simulink model "a1_walking_BM"  (R2022b)
settings: Solver=VariableStepAuto  StartTime=0.0  StopTime=2  RelTol=1e-3
values from neighbouring files (symbols this model uses):
  m = 12    [MPC_Controller.m]    (also in QP_Controller.m; TASK1_rotating_mpc.m; TASK1_walking_backward_mpc.m; TASK1_walking_forward_mpc.m)
  N = 10    [MPC_Controller.m]
undefined symbols (not defined in the file or in its folder): walking_mpc, X, Y, Z
libraries: sm_lib x188, nesl_utility x108
(part 5 of 5)

== system a1_walking_BM/Rear Right Leg/Leg Logger4 ==
  PS-Simulink Converter : nesl_utility/PS-Simulink Converter  PhysicalDomain=network_engine_domain  SubClassName=ps_output  LeftPortType=input  RightPortType=output  PseudoPeriodic=off  Frequencies=[]  VectorFormat=inherit  Unit=inherit  AffineConversion=off
  PS-Simulink Converter1 : nesl_utility/PS-Simulink Converter  PhysicalDomain=network_engine_domain  SubClassName=ps_output  LeftPortType=input  RightPortType=output  PseudoPeriodic=off  Frequencies=[]  VectorFormat=inherit  Unit=inherit  AffineConversion=off
  PS-Simulink Converter2 : nesl_utility/PS-Simulink Converter  PhysicalDomain=network_engine_domain  SubClassName=ps_output  LeftPortType=input  RightPortType=output  PseudoPeriodic=off  Frequencies=[]  VectorFormat=inherit  Unit=inherit  AffineConversion=off
  Scope : Scope  NumInputPorts=3
  angle : PMIOPort  Side=Left
  velocity : PMIOPort  Port=2  Side=Left
  torque : PMIOPort  Port=3  Side=Left
  wires:
  PS-Simulink Converter/1 -> Scope/1  "RR_thigh_joint angle (rad)"
  PS-Simulink Converter2/1 -> Scope/3  "RR_thigh_joint torque (Nm)"
  PS-Simulink Converter1/1 -> Scope/2  "RR_thigh_joint velocity (rad/s)"
  connections:
  PS-Simulink Converter2/LConn1 -- torque/RConn1
  PS-Simulink Converter/LConn1 -- angle/RConn1
  PS-Simulink Converter1/LConn1 -- velocity/RConn1

== system a1_walking_BM/Rear Right Leg/RR_calf ==
  Inertia : sm_lib/Body Elements/Inertia  InertiaType=Custom  Mass=0.166  MassUnits=kg  CenterOfMass=[0, 0, 0]  CenterOfMassUnits=m  MomentsOfInertia=[0.002997972, 0.003014022, 3.2426e-05]  MomentsOfInertiaUnits=kg*m^2  ProductsOfInertia=[0, -0.000141163, 0]  ProductsOfInertiaUnits=kg*m^2  GraphicType=None  MarkerShape=Inertia  MarkerSize=20  GraphicVisPropType=SimpleVisualProperties  GraphicDiffuseColor=[0.5 0.5 0.5]  GraphicSpecularColor=[0.5 0.5 0.5 1.0]  GraphicAmbientColor=[0.15 0.15 0.15 1.0]  GraphicEmissiveColor=[0.0 0.0 0.0 1.0]  GraphicShininess=75  GraphicOpacity=1.0
  InertiaOriginTransform : sm_lib/Frames and Transforms/Rigid Transform  TranslationMethod=Cartesian  TranslationStandardOffset=0  TranslationLengthUnit=m  TranslationStandardAxis=+Z  TranslationCartesianOffset=[0.006435, 0, -0.107388]  TranslationROffset=0  TranslationROffsetUnits=m  TranslationZOffset=0  TranslationZOffsetUnits=m  TranslationThetaOffset=0  TranslationThetaOffsetUnits=deg  RotationMethod=RotationSequence  RotationAngleUnits=deg  RotationStandardAxis=+Z  RotationAngle=0.0  RotationArbitraryAxis=[0 0 1]  FollAlignAxisA=+X  BaseAlignAxisA=+Y  FollAlignAxisB=+Y  BaseAlignAxisB=+Z  RotationSequenceAxes=BaseAxes  RotationSequence=XYZ  RotationSequenceAngles=[0, 0, 0]  RotationSequenceAnglesUnits=rad  RotationMatrix=[1 0 0; 0 1 0; 0 0 1]  Quaternion=[1 0 0 0]
  RR_calf_joint_AxisInvTransform : sm_lib/Frames and Transforms/Rigid Transform  TranslationMethod=Cartesian  TranslationStandardOffset=0  TranslationLengthUnit=m  TranslationStandardAxis=+Z  TranslationCartesianOffset=[0, 0, 0]  TranslationROffset=0  TranslationROffsetUnits=m  TranslationZOffset=0  TranslationZOffsetUnits=m  TranslationThetaOffset=0  TranslationThetaOffsetUnits=deg  RotationMethod=ArbitraryAxis  RotationAngleUnits=rad  RotationStandardAxis=+Z  RotationAngle=1.570796326794897  RotationArbitraryAxis=[-1, 0, 0]  FollAlignAxisA=+X  BaseAlignAxisA=+Y  FollAlignAxisB=+Y  BaseAlignAxisB=+Z  RotationSequenceAxes=FollowerAxes  RotationSequence=XYX  RotationSequenceAngles=[0 0 0]  RotationSequenceAnglesUnits=deg  RotationMatrix=[1 0 0; 0 1 0; 0 0 1]  Quaternion=[1 0 0 0]
  RR_foot_fixed_OriginTransform : sm_lib/Frames and Transforms/Rigid Transform  TranslationMethod=Cartesian  TranslationStandardOffset=0  TranslationLengthUnit=m  TranslationStandardAxis=+Z  TranslationCartesianOffset=[0, 0, -0.2]  TranslationROffset=0  TranslationROffsetUnits=m  TranslationZOffset=0  TranslationZOffsetUnits=m  TranslationThetaOffset=0  TranslationThetaOffsetUnits=deg  RotationMethod=RotationSequence  RotationAngleUnits=deg  RotationStandardAxis=+Z  RotationAngle=0.0  RotationArbitraryAxis=[0 0 1]  FollAlignAxisA=+X  BaseAlignAxisA=+Y  FollAlignAxisB=+Y  BaseAlignAxisB=+Z  RotationSequenceAxes=BaseAxes  RotationSequence=XYZ  RotationSequenceAngles=[0, 0, 0]  RotationSequenceAnglesUnits=rad  RotationMatrix=[1 0 0; 0 1 0; 0 0 1]  Quaternion=[1 0 0 0]
  ReferenceFrame : sm_lib/Frames and Transforms/Reference Frame
  Visual : sm_lib/Body Elements/File Solid  ExtGeomFileName=AME556_project/a1_description/meshes/calf.stl  UnitType=Custom  ExtGeomFileUnits=m  StepReaderType=HEX  ExportConvexHullGeometry=off  InertiaType=Custom  Mass=0  MassUnits=kg  CenterOfMass=[0, 0, 0]  CenterOfMassUnits=m  MomentsOfInertia=[0, 0, 0]  MomentsOfInertiaUnits=kg*m^2  ProductsOfInertia=[0, 0, 0]  ProductsOfInertiaUnits=kg*m^2  BasedOnType=DensityFromFile  Density=1000  DensityUnits=kg/m^3  DoExposeReferenceFrame=on  SerializedFrames=<Frames/>  GraphicType=FromGeometry  MarkerShape=Sphere  MarkerSize=10  GraphicVisPropType=SimpleVisualProperties  GraphicDiffuseColor=[1, 0.423529411765, 0.0392156862745]  GraphicSpecularColor=[0.5 0.5 0.5 1.0]  GraphicAmbientColor=[0.15 0.15 0.15 1.0]  GraphicEmissiveColor=[0.0 0.0 0.0 1.0]  GraphicShininess=75  GraphicOpacity=1
  VisualOriginTransform : sm_lib/Frames and Transforms/Rigid Transform  TranslationMethod=Cartesian  TranslationStandardOffset=0  TranslationLengthUnit=m  TranslationStandardAxis=+Z  TranslationCartesianOffset=[0, 0, 0]  TranslationROffset=0  TranslationROffsetUnits=m  TranslationZOffset=0  TranslationZOffsetUnits=m  TranslationThetaOffset=0  TranslationThetaOffsetUnits=deg  RotationMethod=RotationSequence  RotationAngleUnits=deg  RotationStandardAxis=+Z  RotationAngle=0.0  RotationArbitraryAxis=[0 0 1]  FollAlignAxisA=+X  BaseAlignAxisA=+Y  FollAlignAxisB=+Y  BaseAlignAxisB=+Z  RotationSequenceAxes=BaseAxes  RotationSequence=XYZ  RotationSequenceAngles=[0, 0, 0]  RotationSequenceAnglesUnits=rad  RotationMatrix=[1 0 0; 0 1 0; 0 0 1]  Quaternion=[1 0 0 0]
  F : PMIOPort  Side=Left
  F1 : PMIOPort  Port=2  Side=Right
  connections:
  Inertia/RConn1 -- InertiaOriginTransform/RConn1
  RR_calf_joint_AxisInvTransform/RConn1 -- F/RConn1
  RR_foot_fixed_OriginTransform/RConn1 -- F1/RConn1
  RR_calf_joint_AxisInvTransform/LConn1 -- InertiaOriginTransform/LConn1 -- ReferenceFrame/RConn1 -- VisualOriginTransform/LConn1 -- RR_foot_fixed_OriginTransform/LConn1
  Visual/RConn1 -- VisualOriginTransform/RConn1

== system a1_walking_BM/Rear Right Leg/RR_foot ==
  Inertia : sm_lib/Body Elements/Inertia  InertiaType=Custom  Mass=0.06  MassUnits=kg  CenterOfMass=[0, 0, 0]  CenterOfMassUnits=m  MomentsOfInertia=[9.6e-06, 9.6e-06, 9.6e-06]  MomentsOfInertiaUnits=kg*m^2  ProductsOfInertia=[0, 0, 0]  ProductsOfInertiaUnits=kg*m^2  GraphicType=None  MarkerShape=Inertia  MarkerSize=20  GraphicVisPropType=SimpleVisualProperties  GraphicDiffuseColor=[0.5 0.5 0.5]  GraphicSpecularColor=[0.5 0.5 0.5 1.0]  GraphicAmbientColor=[0.15 0.15 0.15 1.0]  GraphicEmissiveColor=[0.0 0.0 0.0 1.0]  GraphicShininess=75  GraphicOpacity=1.0
  InertiaOriginTransform : sm_lib/Frames and Transforms/Rigid Transform  TranslationMethod=Cartesian  TranslationStandardOffset=0  TranslationLengthUnit=m  TranslationStandardAxis=+Z  TranslationCartesianOffset=[0, 0, 0]  TranslationROffset=0  TranslationROffsetUnits=m  TranslationZOffset=0  TranslationZOffsetUnits=m  TranslationThetaOffset=0  TranslationThetaOffsetUnits=deg  RotationMethod=RotationSequence  RotationAngleUnits=deg  RotationStandardAxis=+Z  RotationAngle=0.0  RotationArbitraryAxis=[0 0 1]  FollAlignAxisA=+X  BaseAlignAxisA=+Y  FollAlignAxisB=+Y  BaseAlignAxisB=+Z  RotationSequenceAxes=BaseAxes  RotationSequence=XYZ  RotationSequenceAngles=[0, 0, 0]  RotationSequenceAnglesUnits=rad  RotationMatrix=[1 0 0; 0 1 0; 0 0 1]  Quaternion=[1 0 0 0]
  ReferenceFrame : sm_lib/Frames and Transforms/Reference Frame
  Visual : sm_lib/Body Elements/Spherical Solid  GraphicAmbientColor=[0.15 0.15 0.15 1.0]  BasedOnType=Density  CenterOfMass=[0, 0, 0]  CenterOfMassUnits=m  GraphicDiffuseColor=[1, 0.423529411765, 0.0392156862745]  Density=1000  DensityUnits=kg/m^3  DoExposeReferenceFrame=on  GraphicEmissiveColor=[0.0 0.0 0.0 1.0]  ExportEntireGeometry=on  SerializedExposedGeometries=<ExposedGeometries><ExposedGeometry><RawGeometryId>entire</RawGeometryId><ExposedGeometryId>G</ExposedGeometryId></ExposedGeometry></ExposedGeometries>  SerializedFrames=<Frames/>  MarkerShape=Sphere  MarkerSize=10  GraphicType=FromGeometry  InertiaType=Custom  Mass=0  MassUnits=kg  MomentsOfInertia=[0, 0, 0]  MomentsOfInertiaUnits=kg*m^2  GraphicOpacity=1  ProductsOfInertia=[0, 0, 0]  ProductsOfInertiaUnits=kg*m^2  GraphicShininess=75  GraphicSpecularColor=[0.5 0.5 0.5 1.0]  SphereRadius=0.01  SphereRadiusUnits=m  GraphicVisPropType=SimpleVisualProperties
  VisualOriginTransform : sm_lib/Frames and Transforms/Rigid Transform  TranslationMethod=Cartesian  TranslationStandardOffset=0  TranslationLengthUnit=m  TranslationStandardAxis=+Z  TranslationCartesianOffset=[0, 0, 0]  TranslationROffset=0  TranslationROffsetUnits=m  TranslationZOffset=0  TranslationZOffsetUnits=m  TranslationThetaOffset=0  TranslationThetaOffsetUnits=deg  RotationMethod=RotationSequence  RotationAngleUnits=deg  RotationStandardAxis=+Z  RotationAngle=0.0  RotationArbitraryAxis=[0 0 1]  FollAlignAxisA=+X  BaseAlignAxisA=+Y  FollAlignAxisB=+Y  BaseAlignAxisB=+Z  RotationSequenceAxes=BaseAxes  RotationSequence=XYZ  RotationSequenceAngles=[0, 0, 0]  RotationSequenceAnglesUnits=rad  RotationMatrix=[1 0 0; 0 1 0; 0 0 1]  Quaternion=[1 0 0 0]
  F : PMIOPort  Side=Left
  G : PMIOPort  Port=2  Side=Left
  connections:
  Inertia/RConn1 -- InertiaOriginTransform/RConn1
  ReferenceFrame/RConn1 -- InertiaOriginTransform/LConn1 -- VisualOriginTransform/LConn1 -- F/RConn1
  Visual/RConn1 -- VisualOriginTransform/RConn1
  G/RConn1 -- Visual/LConn1

== system a1_walking_BM/Rear Right Leg/RR_hip ==
  Inertia : sm_lib/Body Elements/Inertia  InertiaType=Custom  Mass=0.696  MassUnits=kg  CenterOfMass=[0, 0, 0]  CenterOfMassUnits=m  MomentsOfInertia=[0.000469246, 0.00080749, 0.000552929]  MomentsOfInertiaUnits=kg*m^2  ProductsOfInertia=[4.66e-07, 3.42e-07, -9.408999999999999e-06]  ProductsOfInertiaUnits=kg*m^2  GraphicType=None  MarkerShape=Inertia  MarkerSize=20  GraphicVisPropType=SimpleVisualProperties  GraphicDiffuseColor=[0.5 0.5 0.5]  GraphicSpecularColor=[0.5 0.5 0.5 1.0]  GraphicAmbientColor=[0.15 0.15 0.15 1.0]  GraphicEmissiveColor=[0.0 0.0 0.0 1.0]  GraphicShininess=75  GraphicOpacity=1.0
  InertiaOriginTransform : sm_lib/Frames and Transforms/Rigid Transform  TranslationMethod=Cartesian  TranslationStandardOffset=0  TranslationLengthUnit=m  TranslationStandardAxis=+Z  TranslationCartesianOffset=[0.003311, -0.000635, 3.1e-05]  TranslationROffset=0  TranslationROffsetUnits=m  TranslationZOffset=0  TranslationZOffsetUnits=m  TranslationThetaOffset=0  TranslationThetaOffsetUnits=deg  RotationMethod=RotationSequence  RotationAngleUnits=deg  RotationStandardAxis=+Z  RotationAngle=0.0  RotationArbitraryAxis=[0 0 1]  FollAlignAxisA=+X  BaseAlignAxisA=+Y  FollAlignAxisB=+Y  BaseAlignAxisB=+Z  RotationSequenceAxes=BaseAxes  RotationSequence=XYZ  RotationSequenceAngles=[0, 0, 0]  RotationSequenceAnglesUnits=rad  RotationMatrix=[1 0 0; 0 1 0; 0 0 1]  Quaternion=[1 0 0 0]
  RR_hip_fixed_OriginTransform : sm_lib/Frames and Transforms/Rigid Transform  TranslationMethod=Cartesian  TranslationStandardOffset=0  TranslationLengthUnit=m  TranslationStandardAxis=+Z  TranslationCartesianOffset=[0, -0.081, 0]  TranslationROffset=0  TranslationROffsetUnits=m  TranslationZOffset=0  TranslationZOffsetUnits=m  TranslationThetaOffset=0  TranslationThetaOffsetUnits=deg  RotationMethod=RotationSequence  RotationAngleUnits=deg  RotationStandardAxis=+Z  RotationAngle=0.0  RotationArbitraryAxis=[0 0 1]  FollAlignAxisA=+X  BaseAlignAxisA=+Y  FollAlignAxisB=+Y  BaseAlignAxisB=+Z  RotationSequenceAxes=BaseAxes  RotationSequence=XYZ  RotationSequenceAngles=[0, 0, 0]  RotationSequenceAnglesUnits=rad  RotationMatrix=[1 0 0; 0 1 0; 0 0 1]  Quaternion=[1 0 0 0]
  RR_hip_joint_AxisInvTransform : sm_lib/Frames and Transforms/Rigid Transform  TranslationMethod=Cartesian  TranslationStandardOffset=0  TranslationLengthUnit=m  TranslationStandardAxis=+Z  TranslationCartesianOffset=[0, 0, 0]  TranslationROffset=0  TranslationROffsetUnits=m  TranslationZOffset=0  TranslationZOffsetUnits=m  TranslationThetaOffset=0  TranslationThetaOffsetUnits=deg  RotationMethod=ArbitraryAxis  RotationAngleUnits=rad  RotationStandardAxis=+Z  RotationAngle=1.570796326794897  RotationArbitraryAxis=[-0, 1, 0]  FollAlignAxisA=+X  BaseAlignAxisA=+Y  FollAlignAxisB=+Y  BaseAlignAxisB=+Z  RotationSequenceAxes=FollowerAxes  RotationSequence=XYX  RotationSequenceAngles=[0 0 0]  RotationSequenceAnglesUnits=deg  RotationMatrix=[1 0 0; 0 1 0; 0 0 1]  Quaternion=[1 0 0 0]
  RR_thigh_joint_AxisTransform : sm_lib/Frames and Transforms/Rigid Transform  TranslationMethod=Cartesian  TranslationStandardOffset=0  TranslationLengthUnit=m  TranslationStandardAxis=+Z  TranslationCartesianOffset=[0, 0, 0]  TranslationROffset=0  TranslationROffsetUnits=m  TranslationZOffset=0  TranslationZOffsetUnits=m  TranslationThetaOffset=0  TranslationThetaOffsetUnits=deg  RotationMethod=ArbitraryAxis  RotationAngleUnits=rad  RotationStandardAxis=+Z  RotationAngle=1.570796326794897  RotationArbitraryAxis=[-1, 0, 0]  FollAlignAxisA=+X  BaseAlignAxisA=+Y  FollAlignAxisB=+Y  BaseAlignAxisB=+Z  RotationSequenceAxes=FollowerAxes  RotationSequence=XYX  RotationSequenceAngles=[0 0 0]  RotationSequenceAnglesUnits=deg  RotationMatrix=[1 0 0; 0 1 0; 0 0 1]  Quaternion=[1 0 0 0]
  RR_thigh_joint_OriginTransform : sm_lib/Frames and Transforms/Rigid Transform  TranslationMethod=Cartesian  TranslationStandardOffset=0  TranslationLengthUnit=m  TranslationStandardAxis=+Z  TranslationCartesianOffset=[0, -0.0838, 0]  TranslationROffset=0  TranslationROffsetUnits=m  TranslationZOffset=0  TranslationZOffsetUnits=m  TranslationThetaOffset=0  TranslationThetaOffsetUnits=deg  RotationMethod=RotationSequence  RotationAngleUnits=deg  RotationStandardAxis=+Z  RotationAngle=0.0  RotationArbitraryAxis=[0 0 1]  FollAlignAxisA=+X  BaseAlignAxisA=+Y  FollAlignAxisB=+Y  BaseAlignAxisB=+Z  RotationSequenceAxes=BaseAxes  RotationSequence=XYZ  RotationSequenceAngles=[0, 0, 0]  RotationSequenceAnglesUnits=rad  RotationMatrix=[1 0 0; 0 1 0; 0 0 1]  Quaternion=[1 0 0 0]
  ReferenceFrame : sm_lib/Frames and Transforms/Reference Frame
  Visual : sm_lib/Body Elements/File Solid  ExtGeomFileName=AME556_project/a1_description/meshes/hip.stl  UnitType=Custom  ExtGeomFileUnits=m  StepReaderType=HEX  ExportConvexHullGeometry=off  InertiaType=Custom  Mass=0  MassUnits=kg  CenterOfMass=[0, 0, 0]  CenterOfMassUnits=m  MomentsOfInertia=[0, 0, 0]  MomentsOfInertiaUnits=kg*m^2  ProductsOfInertia=[0, 0, 0]  ProductsOfInertiaUnits=kg*m^2  BasedOnType=DensityFromFile  Density=1000  DensityUnits=kg/m^3  DoExposeReferenceFrame=on  SerializedFrames=<Frames/>  GraphicType=FromGeometry  MarkerShape=Sphere  MarkerSize=10  GraphicVisPropType=SimpleVisualProperties  GraphicDiffuseColor=[1, 0.423529411765, 0.0392156862745]  GraphicSpecularColor=[0.5 0.5 0.5 1.0]  GraphicAmbientColor=[0.15 0.15 0.15 1.0]  GraphicEmissiveColor=[0.0 0.0 0.0 1.0]  GraphicShininess=75  GraphicOpacity=1
  VisualOriginTransform : sm_lib/Frames and Transforms/Rigid Transform  TranslationMethod=Cartesian  TranslationStandardOffset=0  TranslationLengthUnit=m  TranslationStandardAxis=+Z  TranslationCartesianOffset=[0, 0, 0]  TranslationROffset=0  TranslationROffsetUnits=m  TranslationZOffset=0  TranslationZOffsetUnits=m  TranslationThetaOffset=0  TranslationThetaOffsetUnits=deg  RotationMethod=RotationSequence  RotationAngleUnits=deg  RotationStandardAxis=+Z  RotationAngle=0.0  RotationArbitraryAxis=[0 0 1]  FollAlignAxisA=+X  BaseAlignAxisA=+Y  FollAlignAxisB=+Y  BaseAlignAxisB=+Z  RotationSequenceAxes=BaseAxes  RotationSequence=XYZ  RotationSequenceAngles=[3.14159265359, 3.14159265359, 0]  RotationSequenceAnglesUnits=rad  RotationMatrix=[1 0 0; 0 1 0; 0 0 1]  Quaternion=[1 0 0 0]
  F : PMIOPort  Side=Left
  F2 : PMIOPort  Port=2  Side=Right
  F1 : PMIOPort  Port=3  Side=Right
  connections:
  Inertia/RConn1 -- InertiaOriginTransform/RConn1
  RR_hip_fixed_OriginTransform/RConn1 -- F1/RConn1
  RR_hip_joint_AxisInvTransform/RConn1 -- F/RConn1
  RR_thigh_joint_AxisTransform/RConn1 -- F2/RConn1
  RR_thigh_joint_AxisTransform/LConn1 -- RR_thigh_joint_OriginTransform/RConn1
  RR_hip_fixed_OriginTransform/LConn1 -- RR_hip_joint_AxisInvTransform/LConn1 -- RR_thigh_joint_OriginTransform/LConn1 -- InertiaOriginTransform/LConn1 -- ReferenceFrame/RConn1 -- VisualOriginTransform/LConn1
  Visual/RConn1 -- VisualOriginTransform/RConn1

== system a1_walking_BM/Rear Right Leg/RR_thigh ==
  Inertia : sm_lib/Body Elements/Inertia  InertiaType=Custom  Mass=1.013  MassUnits=kg  CenterOfMass=[0, 0, 0]  CenterOfMassUnits=m  MomentsOfInertia=[0.005529065, 0.005139339, 0.001367788]  MomentsOfInertiaUnits=kg*m^2  ProductsOfInertia=[-2.2448e-05, 0.000343869, -4.825e-06]  ProductsOfInertiaUnits=kg*m^2  GraphicType=None  MarkerShape=Inertia  MarkerSize=20  GraphicVisPropType=SimpleVisualProperties  GraphicDiffuseColor=[0.5 0.5 0.5]  GraphicSpecularColor=[0.5 0.5 0.5 1.0]  GraphicAmbientColor=[0.15 0.15 0.15 1.0]  GraphicEmissiveColor=[0.0 0.0 0.0 1.0]  GraphicShininess=75  GraphicOpacity=1.0
  InertiaOriginTransform : sm_lib/Frames and Transforms/Rigid Transform  TranslationMethod=Cartesian  TranslationStandardOffset=0  TranslationLengthUnit=m  TranslationStandardAxis=+Z  TranslationCartesianOffset=[-0.003237, 0.022327, -0.027326]  TranslationROffset=0  TranslationROffsetUnits=m  TranslationZOffset=0  TranslationZOffsetUnits=m  TranslationThetaOffset=0  TranslationThetaOffsetUnits=deg  RotationMethod=RotationSequence  RotationAngleUnits=deg  RotationStandardAxis=+Z  RotationAngle=0.0  RotationArbitraryAxis=[0 0 1]  FollAlignAxisA=+X  BaseAlignAxisA=+Y  FollAlignAxisB=+Y  BaseAlignAxisB=+Z  RotationSequenceAxes=BaseAxes  RotationSequence=XYZ  RotationSequenceAngles=[0, 0, 0]  RotationSequenceAnglesUnits=rad  RotationMatrix=[1 0 0; 0 1 0; 0 0 1]  Quaternion=[1 0 0 0]
  RR_calf_joint_AxisTransform : sm_lib/Frames and Transforms/Rigid Transform  TranslationMethod=Cartesian  TranslationStandardOffset=0  TranslationLengthUnit=m  TranslationStandardAxis=+Z  TranslationCartesianOffset=[0, 0, 0]  TranslationROffset=0  TranslationROffsetUnits=m  TranslationZOffset=0  TranslationZOffsetUnits=m  TranslationThetaOffset=0  TranslationThetaOffsetUnits=deg  RotationMethod=ArbitraryAxis  RotationAngleUnits=rad  RotationStandardAxis=+Z  RotationAngle=1.570796326794897  RotationArbitraryAxis=[-1, 0, 0]  FollAlignAxisA=+X  BaseAlignAxisA=+Y  FollAlignAxisB=+Y  BaseAlignAxisB=+Z  RotationSequenceAxes=FollowerAxes  RotationSequence=XYX  RotationSequenceAngles=[0 0 0]  RotationSequenceAnglesUnits=deg  RotationMatrix=[1 0 0; 0 1 0; 0 0 1]  Quaternion=[1 0 0 0]
  RR_calf_joint_OriginTransform : sm_lib/Frames and Transforms/Rigid Transform  TranslationMethod=Cartesian  TranslationStandardOffset=0  TranslationLengthUnit=m  TranslationStandardAxis=+Z  TranslationCartesianOffset=[0, 0, -0.2]  TranslationROffset=0  TranslationROffsetUnits=m  TranslationZOffset=0  TranslationZOffsetUnits=m  TranslationThetaOffset=0  TranslationThetaOffsetUnits=deg  RotationMethod=RotationSequence  RotationAngleUnits=deg  RotationStandardAxis=+Z  RotationAngle=0.0  RotationArbitraryAxis=[0 0 1]  FollAlignAxisA=+X  BaseAlignAxisA=+Y  FollAlignAxisB=+Y  BaseAlignAxisB=+Z  RotationSequenceAxes=BaseAxes  RotationSequence=XYZ  RotationSequenceAngles=[0, 0, 0]  RotationSequenceAnglesUnits=rad  RotationMatrix=[1 0 0; 0 1 0; 0 0 1]  Quaternion=[1 0 0 0]
  RR_thigh_joint_AxisInvTransform : sm_lib/Frames and Transforms/Rigid Transform  TranslationMethod=Cartesian  TranslationStandardOffset=0  TranslationLengthUnit=m  TranslationStandardAxis=+Z  TranslationCartesianOffset=[0, 0, 0]  TranslationROffset=0  TranslationROffsetUnits=m  TranslationZOffset=0  TranslationZOffsetUnits=m  TranslationThetaOffset=0  TranslationThetaOffsetUnits=deg  RotationMethod=ArbitraryAxis  RotationAngleUnits=rad  RotationStandardAxis=+Z  RotationAngle=1.570796326794897  RotationArbitraryAxis=[-1, 0, 0]  FollAlignAxisA=+X  BaseAlignAxisA=+Y  FollAlignAxisB=+Y  BaseAlignAxisB=+Z  RotationSequenceAxes=FollowerAxes  RotationSequence=XYX  RotationSequenceAngles=[0 0 0]  RotationSequenceAnglesUnits=deg  RotationMatrix=[1 0 0; 0 1 0; 0 0 1]  Quaternion=[1 0 0 0]
  ReferenceFrame : sm_lib/Frames and Transforms/Reference Frame
  Visual : sm_lib/Body Elements/File Solid  ExtGeomFileName=AME556_project/a1_description/meshes/thigh_mirror.stl  UnitType=Custom  ExtGeomFileUnits=m  StepReaderType=HEX  ExportConvexHullGeometry=on  InertiaType=Custom  Mass=0  MassUnits=kg  CenterOfMass=[0, 0, 0]  CenterOfMassUnits=m  MomentsOfInertia=[0, 0, 0]  MomentsOfInertiaUnits=kg*m^2  ProductsOfInertia=[0, 0, 0]  ProductsOfInertiaUnits=kg*m^2  BasedOnType=DensityFromFile  Density=1000  DensityUnits=kg/m^3  DoExposeReferenceFrame=on  SerializedFrames=<Frames/>  GraphicType=FromGeometry  MarkerShape=Sphere  MarkerSize=10  GraphicVisPropType=SimpleVisualProperties  GraphicDiffuseColor=[1, 0.423529411765, 0.0392156862745]  GraphicSpecularColor=[0.5 0.5 0.5 1.0]  GraphicAmbientColor=[0.15 0.15 0.15 1.0]  GraphicEmissiveColor=[0.0 0.0 0.0 1.0]  GraphicShininess=75  GraphicOpacity=1
  VisualOriginTransform : sm_lib/Frames and Transforms/Rigid Transform  TranslationMethod=Cartesian  TranslationStandardOffset=0  TranslationLengthUnit=m  TranslationStandardAxis=+Z  TranslationCartesianOffset=[0, 0, 0]  TranslationROffset=0  TranslationROffsetUnits=m  TranslationZOffset=0  TranslationZOffsetUnits=m  TranslationThetaOffset=0  TranslationThetaOffsetUnits=deg  RotationMethod=RotationSequence  RotationAngleUnits=deg  RotationStandardAxis=+Z  RotationAngle=0.0  RotationArbitraryAxis=[0 0 1]  FollAlignAxisA=+X  BaseAlignAxisA=+Y  FollAlignAxisB=+Y  BaseAlignAxisB=+Z  RotationSequenceAxes=BaseAxes  RotationSequence=XYZ  RotationSequenceAngles=[0, 0, 0]  RotationSequenceAnglesUnits=rad  RotationMatrix=[1 0 0; 0 1 0; 0 0 1]  Quaternion=[1 0 0 0]
  F : PMIOPort  Side=Left
  G : PMIOPort  Port=2  Side=Right
  F1 : PMIOPort  Port=3  Side=Right
  connections:
  Inertia/RConn1 -- InertiaOriginTransform/RConn1
  RR_calf_joint_AxisTransform/RConn1 -- F1/RConn1
  RR_calf_joint_AxisTransform/LConn1 -- RR_calf_joint_OriginTransform/RConn1
  RR_thigh_joint_AxisInvTransform/RConn1 -- F/RConn1
  RR_calf_joint_OriginTransform/LConn1 -- InertiaOriginTransform/LConn1 -- ReferenceFrame/RConn1 -- VisualOriginTransform/LConn1 -- RR_thigh_joint_AxisInvTransform/LConn1
  Visual/RConn1 -- VisualOriginTransform/RConn1
  G/RConn1 -- Visual/LConn1

== system a1_walking_BM/Rear Right Leg/RR_thigh_shoulder ==
  ReferenceFrame : sm_lib/Frames and Transforms/Reference Frame
  F : PMIOPort  Side=Left
  connections:
  ReferenceFrame/RConn1 -- F/RConn1

== system a1_walking_BM/Stand Controller/Subsystem1 ==
  angle : Inport
  velocity : Inport  Port=2
  Add : Sum
  Constant1 : Constant  Value=-2
  Constant2 : Constant  Value=-20
  Constant3 : Constant  Value=0.5
  Product : Product
  Product1 : Product
  Saturation : Saturate  UpperLimit=33.5  LowerLimit=-33.5
  Subtract : Sum  Inputs=+-
  Torque : Outport
  wires:
  angle/1 -> Subtract/1
  Constant2/1 -> Product/2
  Subtract/1 -> Product/1
  Constant1/1 -> Product1/2
  velocity/1 -> Product1/1
  Product1/1 -> Add/2
  Product/1 -> Add/1
  Constant3/1 -> Subtract/2
  Add/1 -> Saturation/1
  Saturation/1 -> Torque/1

== system a1_walking_BM/Stand Controller/Subsystem10 ==
  angle : Inport
  velocity : Inport  Port=2
  Add : Sum
  Constant1 : Constant  Value=-6
  Constant2 : Constant  Value=-60
  Constant3 : Constant  Value=0.8
  Product : Product
  Product1 : Product
  Saturation : Saturate  UpperLimit=33.5  LowerLimit=-33.5
  Subtract : Sum  Inputs=+-
  Torque : Outport
  wires:
  angle/1 -> Subtract/1
  Constant2/1 -> Product/2
  Subtract/1 -> Product/1
  Constant1/1 -> Product1/2
  velocity/1 -> Product1/1
  Product1/1 -> Add/2
  Product/1 -> Add/1
  Constant3/1 -> Subtract/2
  Add/1 -> Saturation/1
  Saturation/1 -> Torque/1

== system a1_walking_BM/Stand Controller/Subsystem11 ==
  angle : Inport
  velocity : Inport  Port=2
  Add : Sum
  Constant1 : Constant  Value=-4
  Constant2 : Constant  Value=-40
  Constant3 : Constant  Value=-1
  Product : Product
  Product1 : Product
  Saturation : Saturate  UpperLimit=33.5  LowerLimit=-33.5
  Subtract : Sum  Inputs=+-
  Torque : Outport
  wires:
  angle/1 -> Subtract/1
  Constant2/1 -> Product/2
  Subtract/1 -> Product/1
  Constant1/1 -> Product1/2
  velocity/1 -> Product1/1
  Product1/1 -> Add/2
  Product/1 -> Add/1
  Constant3/1 -> Subtract/2
  Add/1 -> Saturation/1
  Saturation/1 -> Torque/1

== system a1_walking_BM/Stand Controller/Subsystem12 ==
  angle : Inport
  velocity : Inport  Port=2
  Add : Sum
  Constant1 : Constant  Value=-2
  Constant2 : Constant  Value=-20
  Constant3 : Constant  Value=0
  Product : Product
  Product1 : Product
  Saturation : Saturate  UpperLimit=33.5  LowerLimit=-33.5
  Subtract : Sum  Inputs=+-
  Torque : Outport
  wires:
  angle/1 -> Subtract/1
  Constant2/1 -> Product/2
  Subtract/1 -> Product/1
  Constant1/1 -> Product1/2
  velocity/1 -> Product1/1
  Product1/1 -> Add/2
  Product/1 -> Add/1
  Constant3/1 -> Subtract/2
  Add/1 -> Saturation/1
  Saturation/1 -> Torque/1

== system a1_walking_BM/Stand Controller/Subsystem2 ==
  angle : Inport
  velocity : Inport  Port=2
  Add : Sum
  Constant1 : Constant  Value=-6
  Constant2 : Constant  Value=-60
  Constant3 : Constant  Value=0.8
  Product : Product
  Product1 : Product
  Saturation : Saturate  UpperLimit=33.5  LowerLimit=-33.5
  Subtract : Sum  Inputs=+-
  Torque : Outport
  wires:
  angle/1 -> Subtract/1
  Constant2/1 -> Product/2
  Subtract/1 -> Product/1
  Constant1/1 -> Product1/2
  velocity/1 -> Product1/1
  Product1/1 -> Add/2
  Product/1 -> Add/1
  Constant3/1 -> Subtract/2
  Add/1 -> Saturation/1
  Saturation/1 -> Torque/1

== system a1_walking_BM/Stand Controller/Subsystem3 ==
  angle : Inport
  velocity : Inport  Port=2
  Add : Sum
  Constant1 : Constant  Value=-2
  Constant2 : Constant  Value=-20
  Constant3 : Constant  Value=-1
  Product : Product
  Product1 : Product
  Saturation : Saturate  UpperLimit=33.5  LowerLimit=-33.5
  Subtract : Sum  Inputs=+-
  Torque : Outport
  wires:
  angle/1 -> Subtract/1
  Constant2/1 -> Product/2
  Subtract/1 -> Product/1
  Constant1/1 -> Product1/2
  velocity/1 -> Product1/1
  Product1/1 -> Add/2
  Product/1 -> Add/1
  Constant3/1 -> Subtract/2
  Add/1 -> Saturation/1
  Saturation/1 -> Torque/1

== system a1_walking_BM/Stand Controller/Subsystem4 ==
  angle : Inport
  velocity : Inport  Port=2
  Add : Sum
  Constant1 : Constant  Value=-4
  Constant2 : Constant  Value=-40
  Constant3 : Constant  Value=-1
  Product : Product
  Product1 : Product
  Saturation : Saturate  UpperLimit=33.5  LowerLimit=-33.5
  Subtract : Sum  Inputs=+-
  Torque : Outport
  wires:
  angle/1 -> Subtract/1
  Constant2/1 -> Product/2
  Subtract/1 -> Product/1
  Constant1/1 -> Product1/2
  velocity/1 -> Product1/1
  Product1/1 -> Add/2
  Product/1 -> Add/1
  Constant3/1 -> Subtract/2
  Add/1 -> Saturation/1
  Saturation/1 -> Torque/1

== system a1_walking_BM/Stand Controller/Subsystem5 ==
  angle : Inport
  velocity : Inport  Port=2
  Add : Sum
  Constant1 : Constant  Value=-0.5
  Constant2 : Constant  Value=-5
  Constant3 : Constant  Value=0
  Product : Product
  Product1 : Product
  Saturation : Saturate  UpperLimit=33.5  LowerLimit=-33.5
  Subtract : Sum  Inputs=+-
  Torque : Outport
  wires:
  angle/1 -> Subtract/1
  Constant2/1 -> Product/2
  Subtract/1 -> Product/1
  Constant1/1 -> Product1/2
  velocity/1 -> Product1/1
  Product1/1 -> Add/2
  Product/1 -> Add/1
  Constant3/1 -> Subtract/2
  Add/1 -> Saturation/1
  Saturation/1 -> Torque/1

== system a1_walking_BM/Stand Controller/Subsystem6 ==
  angle : Inport
  velocity : Inport  Port=2
  Add : Sum
  Constant1 : Constant  Value=-2
  Constant2 : Constant  Value=-20
  Constant3 : Constant  Value=0
  Product : Product
  Product1 : Product
  Saturation : Saturate  UpperLimit=33.5  LowerLimit=-33.5
  Subtract : Sum  Inputs=+-
  Torque : Outport
  wires:
  angle/1 -> Subtract/1
  Constant2/1 -> Product/2
  Subtract/1 -> Product/1
  Constant1/1 -> Product1/2
  velocity/1 -> Product1/1
  Product1/1 -> Add/2
  Product/1 -> Add/1
  Constant3/1 -> Subtract/2
  Add/1 -> Saturation/1
  Saturation/1 -> Torque/1

== system a1_walking_BM/Stand Controller/Subsystem7 ==
  angle : Inport
  velocity : Inport  Port=2
  Add : Sum
  Constant1 : Constant  Value=-2
  Constant2 : Constant  Value=-20
  Constant3 : Constant  Value=0.5
  Product : Product
  Product1 : Product
  Saturation : Saturate  UpperLimit=33.5  LowerLimit=-33.5
  Subtract : Sum  Inputs=+-
  Torque : Outport
  wires:
  angle/1 -> Subtract/1
  Constant2/1 -> Product/2
  Subtract/1 -> Product/1
  Constant1/1 -> Product1/2
  velocity/1 -> Product1/1
  Product1/1 -> Add/2
  Product/1 -> Add/1
  Constant3/1 -> Subtract/2
  Add/1 -> Saturation/1
  Saturation/1 -> Torque/1

== system a1_walking_BM/Stand Controller/Subsystem8 ==
  angle : Inport
  velocity : Inport  Port=2
  Add : Sum
  Constant1 : Constant  Value=-2
  Constant2 : Constant  Value=-20
  Constant3 : Constant  Value=-1
  Product : Product
  Product1 : Product
  Saturation : Saturate  UpperLimit=33.5  LowerLimit=-33.5
  Subtract : Sum  Inputs=+-
  Torque : Outport
  wires:
  angle/1 -> Subtract/1
  Constant2/1 -> Product/2
  Subtract/1 -> Product/1
  Constant1/1 -> Product1/2
  velocity/1 -> Product1/1
  Product1/1 -> Add/2
  Product/1 -> Add/1
  Constant3/1 -> Subtract/2
  Add/1 -> Saturation/1
  Saturation/1 -> Torque/1

== system a1_walking_BM/Stand Controller/Subsystem9 ==
  angle : Inport
  velocity : Inport  Port=2
  Add : Sum
  Constant1 : Constant  Value=-0.5
  Constant2 : Constant  Value=-5
  Constant3 : Constant  Value=0
  Product : Product
  Product1 : Product
  Saturation : Saturate  UpperLimit=33.5  LowerLimit=-33.5
  Subtract : Sum  Inputs=+-
  Torque : Outport
  wires:
  angle/1 -> Subtract/1
  Constant2/1 -> Product/2
  Subtract/1 -> Product/1
  Constant1/1 -> Product1/2
  velocity/1 -> Product1/1
  Product1/1 -> Add/2
  Product/1 -> Add/1
  Constant3/1 -> Subtract/2
  Add/1 -> Saturation/1
  Saturation/1 -> Torque/1

== matlab function a1_walking_BM/Stand Controller/MATLAB Function4 ==
  data: angle_vector input; hip_angle output; thigh_angle output; calf_angle output
function [hip_angle, thigh_angle, calf_angle] = fcn(angle_vector)

hip_angle = angle_vector(1);
thigh_angle = angle_vector(2);
calf_angle = angle_vector(3);

== matlab function a1_walking_BM/Stand Controller/MATLAB Function5 ==
  data: velocity_vector input; hip_velocity output; thigh_velocity output; calf_velocity output
function [hip_velocity, thigh_velocity, calf_velocity] = fcn(velocity_vector)

hip_velocity = velocity_vector(1);
thigh_velocity = velocity_vector(2);
calf_velocity = velocity_vector(3);

== matlab function a1_walking_BM/Stand Controller/MATLAB Function6 ==
  data: angle_vector input; hip_angle output; thigh_angle output; calf_angle output
function [hip_angle, thigh_angle, calf_angle] = fcn(angle_vector)

hip_angle = angle_vector(1);
thigh_angle = angle_vector(2);
calf_angle = angle_vector(3);

== matlab function a1_walking_BM/Stand Controller/MATLAB Function7 ==
  data: velocity_vector input; hip_velocity output; thigh_velocity output; calf_velocity output
function [hip_velocity, thigh_velocity, calf_velocity] = fcn(velocity_vector)

hip_velocity = velocity_vector(1);
thigh_velocity = velocity_vector(2);
calf_velocity = velocity_vector(3);

== matlab function a1_walking_BM/Swing Controller/MATLAB Function ==
  data: v_com_vec input; F output; t input; T_stance input; v_desired input; p_hip input
function F = fcn(v_com_vec,t,T_stance,v_desired,p_hip)


%% NOTE - THIS CODE IS NOT COMPLETE YET
% Find K_step - this value can be tuned with z_com_desired
z_com_desired = 0.1;
g = 9.81;
K_step = sqrt(z_com_desired/g);

% Find P_foot_desired
p_foot_desired = p_hip+(T_stance/2)*v_com_vec+K_step*(v_com_vec-v_desired);

% Find F_swing
Kp = 1; 
Kd = 1; 
F_swing = Kp*(p_foot_desired-p_foot)+Kd*(foot_vel_desired-foot_vel)

F = v_com_vec;

== matlab function a1_walking_BM/Convert Forces to Torque/Force to Torque ==
  data: F input; Tau_RR output; RR_ang_vec input; RL_ang_vec input; FL_ang_vec input; FR_ang_vec input; Tau_FR output; Tau_FL output; Tau_RL output
function [Tau_RR,Tau_FR,Tau_FL,Tau_RL]= fcn(F,RR_ang_vec,RL_ang_vec,FL_ang_vec,FR_ang_vec)
    % TODO - Convert forces to torques using the inverse jacobian

    %% NOTE - The inverse jacobians were calculated by finding the end
    % effector position and taking the partial with respect to each joint
    % Theta 2 is the hip angle 
    % Theta 4 is the thigh angle
    % Theta 5 is the calf angle 
    a2 = 0.0838; %This is the hip length (m)
    a4 = 0.2; %This is the thigh length (m)
    a5 = 0.2; %This is the calf length (m)

    % Get forces from the force vector 
    % NOTE - VERIFY THAT THESE ARE THE CORRECT VECTORS (I am unsure)
    F_FL = F(1:3);
    F_FR = F(4:6);
    F_RL = F(7:9);
    F_RR = F(10:12);

    %% Calculate the force for the RR leg - NOTE: The right legs have the
    % same jacobians
    theta2 = RR_ang_vec(1); % RE-Define theta 2 
    theta4 = RR_ang_vec(2); % RE-Define theta 4
    theta5 = RR_ang_vec(3); % RE-Define theta 5
    inJ_R_RR = [                                                                       0, a2*sin(theta2) + a4*cos(theta2)*cos(theta4) + a5*cos(theta2)*cos(theta4)*cos(theta5) - a5*cos(theta2)*sin(theta4)*sin(theta5), a4*cos(theta4)*sin(theta2) - a2*cos(theta2) + a5*cos(theta4)*cos(theta5)*sin(theta2) - a5*sin(theta2)*sin(theta4)*sin(theta5);
    a5*sin(theta4)*sin(theta5) - a5*cos(theta4)*cos(theta5) - a4*cos(theta4),                - a4*sin(theta2)*sin(theta4) - a5*cos(theta4)*sin(theta2)*sin(theta5) - a5*cos(theta5)*sin(theta2)*sin(theta4),                  a4*cos(theta2)*sin(theta4) + a5*cos(theta2)*cos(theta4)*sin(theta5) + a5*cos(theta2)*cos(theta5)*sin(theta4);
                     a5*sin(theta4)*sin(theta5) - a5*cos(theta4)*cos(theta5),                                             - a5*cos(theta4)*sin(theta2)*sin(theta5) - a5*cos(theta5)*sin(theta2)*sin(theta4),                                               a5*cos(theta2)*cos(theta4)*sin(theta5) + a5*cos(theta2)*cos(theta5)*sin(theta4)];
     
    Tau_RR = -inJ_R_RR*F_RR;

    %% Calculate the force for the FR leg - NOTE: The right legs have the
    % same jacobians
    theta2 = FR_ang_vec(1); % RE-Define theta 2 
    theta4 = FR_ang_vec(2); % RE-Define theta 4
    theta5 = FR_ang_vec(3); % RE-Define theta 5
    inJ_R_FR = [                                                                       0, a2*sin(theta2) + a4*cos(theta2)*cos(theta4) + a5*cos(theta2)*cos(theta4)*cos(theta5) - a5*cos(theta2)*sin(theta4)*sin(theta5), a4*cos(theta4)*sin(theta2) - a2*cos(theta2) + a5*cos(theta4)*cos(theta5)*sin(theta2) - a5*sin(theta2)*sin(theta4)*sin(theta5);
    a5*sin(theta4)*sin(theta5) - a5*cos(theta4)*cos(theta5) - a4*cos(theta4),                - a4*sin(theta2)*sin(theta4) - a5*cos(theta4)*sin(theta2)*sin(theta5) - a5*cos(theta5)*sin(theta2)*sin(theta4),                  a4*cos(theta2)*sin(theta4) + a5*cos(theta2)*cos(theta4)*sin(theta5) + a5*cos(theta2)*cos(theta5)*sin(theta4);
                     a5*sin(theta4)*sin(theta5) - a5*cos(theta4)*cos(theta5),                                             - a5*cos(theta4)*sin(theta2)*sin(theta5) - a5*cos(theta5)*sin(theta2)*sin(theta4),                                               a5*cos(theta2)*cos(theta4)*sin(theta5) + a5*cos(theta2)*cos(theta5)*sin(theta4)];
     
    Tau_FR = -inJ_R_FR*F_FR;

    %% Calculate the force for the FL leg - NOTE: The right legs have the
    % same jacobians
    theta2 = FL_ang_vec(1); % RE-Define theta 2 
    theta4 = FL_ang_vec(2); % RE-Define theta 4
    theta5 = FL_ang_vec(3); % RE-Define theta 5
    inJ_L_FL = [                                                                       0, a4*cos(theta2)*cos(theta4) - a2*sin(theta2) + a5*cos(theta2)*cos(theta4)*cos(theta5) - a5*cos(theta2)*sin(theta4)*sin(theta5), a2*cos(theta2) + a4*cos(theta4)*sin(theta2) + a5*cos(theta4)*cos(theta5)*sin(theta2) - a5*sin(theta2)*sin(theta4)*sin(theta5);
    a5*sin(theta4)*sin(theta5) - a5*cos(theta4)*cos(theta5) - a4*cos(theta4),                - a4*sin(theta2)*sin(theta4) - a5*cos(theta4)*sin(theta2)*sin(theta5) - a5*cos(theta5)*sin(theta2)*sin(theta4),                  a4*cos(theta2)*sin(theta4) + a5*cos(theta2)*cos(theta4)*sin(theta5) + a5*cos(theta2)*cos(theta5)*sin(theta4);
                     a5*sin(theta4)*sin(theta5) - a5*cos(theta4)*cos(theta5),                                             - a5*cos(theta4)*sin(theta2)*sin(theta5) - a5*cos(theta5)*sin(theta2)*sin(theta4),                                               a5*cos(theta2)*cos(theta4)*sin(theta5) + a5*cos(theta2)*cos(theta5)*sin(theta4)];
     
    Tau_FL = -inJ_L_FL*F_FL;


    %% Calculate the force for the RL leg - NOTE: The right legs have the
    % same jacobians
    theta2 = RL_ang_vec(1); % RE-Define theta 2 
    theta4 = RL_ang_vec(2); % RE-Define theta 4
    theta5 = RL_ang_vec(3); % RE-Define theta 5
    inJ_L_RL = [                                                                       0, a4*cos(theta2)*cos(theta4) - a2*sin(theta2) + a5*cos(theta2)*cos(theta4)*cos(theta5) - a5*cos(theta2)*sin(theta4)*sin(theta5), a2*cos(theta2) + a4*cos(theta4)*sin(theta2) + a5*cos(theta4)*cos(theta5)*sin(theta2) - a5*sin(theta2)*sin(theta4)*sin(theta5);
    a5*sin(theta4)*sin(theta5) - a5*cos(theta4)*cos(theta5) - a4*cos(theta4),                - a4*sin(theta2)*sin(theta4) - a5*cos(theta4)*sin(theta2)*sin(theta5) - a5*cos(theta5)*sin(theta2)*sin(theta4),                  a4*cos(theta2)*sin(theta4) + a5*cos(theta2)*cos(theta4)*sin(theta5) + a5*cos(theta2)*cos(theta5)*sin(theta4);
                     a5*sin(theta4)*sin(theta5) - a5*cos(theta4)*cos(theta5),                                             - a5*cos(theta4)*sin(theta2)*sin(theta5) - a5*cos(theta5)*sin(theta2)*sin(theta4),                                               a5*cos(theta2)*cos(theta4)*sin(theta5) + a5*cos(theta2)*cos(theta5)*sin(theta4)];
     
    Tau_RL = -inJ_L_RL*F_RL;

== matlab function a1_walking_BM/Rigid Body Controller/Rotation Matrix to Eul ==
  data: u input; y output
function y = fcn(u)
y = rotm2eul(u);

== matlab function a1_walking_BM/Rear Left Leg/Separate Torques ==
  data: torque_vector input; hip_torque output; thigh_torque output; calf_torque output
function [hip_torque, thigh_torque, calf_torque] = fcn(torque_vector)

hip_torque = torque_vector(1);
thigh_torque = torque_vector(2);
calf_torque = torque_vector(3);

== matlab function a1_walking_BM/Front Right Leg/Separate Torques ==
  data: torque_vector input; hip_torque output; thigh_torque output; calf_torque output
function [hip_torque, thigh_torque, calf_torque] = fcn(torque_vector)

hip_torque = torque_vector(1);
thigh_torque = torque_vector(2);
calf_torque = torque_vector(3);

== matlab function a1_walking_BM/Rear Right Leg/Separate Torques ==
  data: torque_vector input; hip_torque output; thigh_torque output; calf_torque output
function [hip_torque, thigh_torque, calf_torque] = fcn(torque_vector)

hip_torque = torque_vector(1);
thigh_torque = torque_vector(2);
calf_torque = torque_vector(3);

== matlab function a1_walking_BM/Front Left Leg/Separate Torques ==
  data: torque_vector input; hip_torque output; thigh_torque output; calf_torque output
function [hip_torque, thigh_torque, calf_torque] = fcn(torque_vector)

hip_torque = torque_vector(1);
thigh_torque = torque_vector(2);
calf_torque = torque_vector(3);

== matlab function a1_walking_BM/Stand Controller/MATLAB Function ==
  data: angle_vector input; hip_angle output; thigh_angle output; calf_angle output
function [hip_angle, thigh_angle, calf_angle] = fcn(angle_vector)

hip_angle = angle_vector(1);
thigh_angle = angle_vector(2);
calf_angle = angle_vector(3);

== matlab function a1_walking_BM/Stand Controller/MATLAB Function1 ==
  data: velocity_vector input; hip_velocity output; thigh_velocity output; calf_velocity output
function [hip_velocity, thigh_velocity, calf_velocity] = fcn(velocity_vector)

hip_velocity = velocity_vector(1);
thigh_velocity = velocity_vector(2);
calf_velocity = velocity_vector(3);

== matlab function a1_walking_BM/Stand Controller/MATLAB Function2 ==
  data: angle_vector input; hip_angle output; thigh_angle output; calf_angle output
function [hip_angle, thigh_angle, calf_angle] = fcn(angle_vector)

hip_angle = angle_vector(1);
thigh_angle = angle_vector(2);
calf_angle = angle_vector(3);

== matlab function a1_walking_BM/Stand Controller/MATLAB Function3 ==
  data: velocity_vector input; hip_velocity output; thigh_velocity output; calf_velocity output
function [hip_velocity, thigh_velocity, calf_velocity] = fcn(velocity_vector)

hip_velocity = velocity_vector(1);
thigh_velocity = velocity_vector(2);
calf_velocity = velocity_vector(3);
